simulink model "Observer_hoeksnelheidsmeter_SIU1"  (R2018b)
settings: Solver=FixedStepAuto  StartTime=0.0  StopTime=2  RelTol=1e-3
values from neighbouring files (symbols this model uses):
  A = [-(bm*(n^2) + bg)/(Jm*(n^2) + Jg) Kt*n/(Jm*(n^2) + Jg) ... (first row only)    [integratieTestScript.m]    (also in integratieTestScriptSIU2.m)
  B = [0 ... (first row only)    [integratieTestScript.m]    (also in integratieTestScriptSIU2.m)
  C = [1 0]    [integratieTestScript.m]    (also in integratieTestScriptSIU2.m)
  D = [0]    [integratieTestScript.m]    (also in integratieTestScriptSIU2.m)
  Kt = 0.083796    [integratieTestScript.m]
  n = 16.5    [integratieTestScript.m]
undefined symbols (not defined in the file or in its folder): DiscIntNeverNeededParam
libraries: simulink x2, dspswit3 x2, dspstat3 x1, peLuenbergerObserver x1, pePwmGenerator x1, powerlib_meascontrol x1
settings Model: Creator=Roberto  LastModifiedBy=Roberto

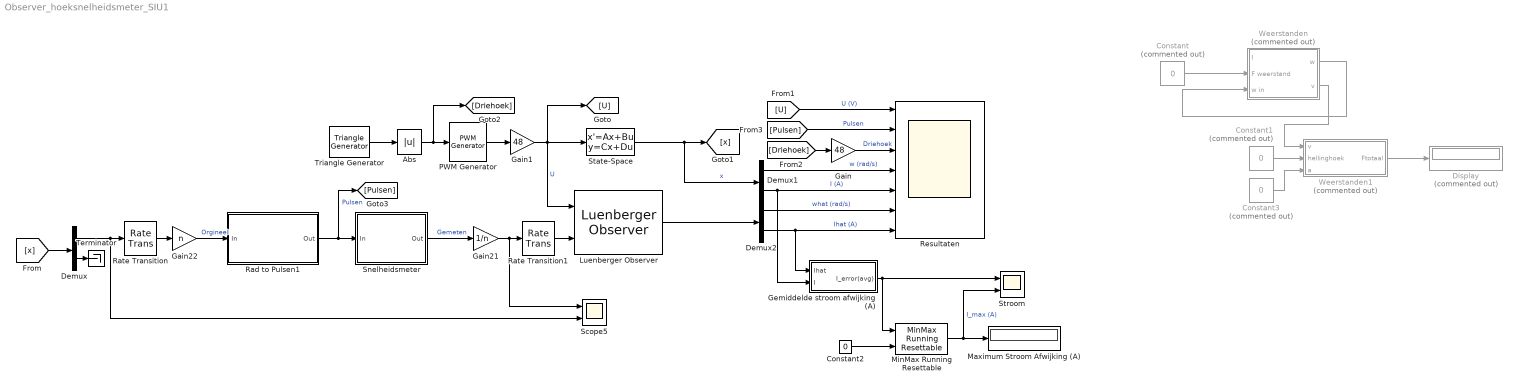
== system Observer_hoeksnelheidsmeter_SIU1 ==
  Abs : Abs
  Constant : Constant  Commented=on  Value=0
  Constant1 : Constant  Commented=on  Value=0
  Constant2 : Constant  Value=0
  Constant3 : Constant  Commented=on  Value=0
  Demux : Demux  Outputs=2
  Demux1 : Demux  Outputs=2
  Demux2 : Demux  Outputs=2
  Display : Display  Commented=on
  Gain : Gain  Gain=48
  Gain1 : Gain  Gain=48
  Gain21 : Gain  Gain=1/n
  Gain22 : Gain  Gain=n
  Gemiddelde stroom afwijking (A) : Subsystem
  Luenberger Observer : peLuenbergerObserver/Luenberger Observer  StateSpaceType=Continuous-time  Ad=Adh  Bd=Bdh  Cd=C  Dd=0  A=A  B=B  C=C  D=D  ObserverDesign=Observer gain  Ld=L  DesiredEigenvalues=eigenVal  x0=[0 0]  Tsd=0.1  Ts=1e-6
  Maximum Stroom Afwijking (A) : Display
  MinMax Running Resettable : simulink/Math Operations/MinMax Running Resettable  Function=max  vinit=0.0
  PWM Generator : pePwmGenerator/PWM Generator  CarrCount=Up  Tper=1/20000  Ts=1e-6
  Rad to Pulsen1 : Subsystem
  Rate Transition : RateTransition  OutPortSampleTime=1/100000
  Rate Transition1 : RateTransition  OutPortSampleTime=1e-6
  Resultaten : Scope  NumInputPorts=7
  Scope5 : Scope  NumInputPorts=2
  Snelheidsmeter : Subsystem
  State-Space : StateSpace  A=A  B=B  C=eye(2)  D=[0; 0]  InitialCondition=0
  Stroom : Scope  NumInputPorts=2
  Terminator : Terminator
  Triangle Generator : powerlib_meascontrol/Pulse & Signal Generators/Triangle Generator  Freq=0.5  Phase=90  Ts=1e-6
  Weerstanden : Subsystem  Commented=on
  Weerstanden1 : Subsystem  Commented=on
      mask init:
      | %% Parameter
      | 
      | %Mass'a
      | 
      | m = 2.067%130
      | 
      | g = 9.81
      | 
      | frol = 0.005
  wires:
  State-Space/1 -> Demux1/1, [x]  "x"
  Luenberger Observer/1 -> Demux2/1
  Gain22/1 -> Rad to Pulsen1/1(In)  "Orgineel"
  Snelheidsmeter/1(Out) -> Gain21/1  "Gemeten"
  Rad to Pulsen1/1(Out) -> [Pulsen], Snelheidsmeter/1(In)  "Pulsen"
  Demux/1 -> Scope5/2, Rate Transition/1
  Gain21/1 -> Scope5/1, Rate Transition1/1
  Rate Transition/1 -> Gain22/1
  Constant/1 -> Weerstanden/2(F weerstand)
  Weerstanden/1(w) -> Weerstanden/3(w in)
  Constant3/1 -> Weerstanden1/3(a)
  Constant1/1 -> Weerstanden1/2(hellinghoek)
  Weerstanden1/1(Ftotaal) -> Display/1
  Weerstanden/2(v) -> Weerstanden1/1(v)
  Rate Transition1/1 -> Luenberger Observer/2
  [x] -> Demux/1
  Demux/2 -> Terminator/1
  Constant2/1 -> MinMax Running Resettable/2
  MinMax Running Resettable/1 -> Stroom/2, Maximum Stroom Afwijking (A)/1  "I_max (A)"
  Gain/1 -> Resultaten/3  "Driehoek"
  [U] -> Resultaten/1  "U (V)"
  Demux2/1 -> Resultaten/6  "what (rad/s)"
  Demux2/2 -> Gemiddelde stroom afwijking (A)/1(Ihat), Resultaten/7  "Ihat (A)"
  [Driehoek] -> Gain/1
  Demux1/1 -> Resultaten/4  "w (rad/s)"
  Demux1/2 -> Gemiddelde stroom afwijking (A)/2(I), Resultaten/5  "I (A)"
  Gemiddelde stroom afwijking (A)/1(I_error(avg)) -> Stroom/1, MinMax Running Resettable/1
  Triangle Generator/1 -> Abs/1
  Abs/1 -> [Driehoek], PWM Generator/1
  Gain1/1 -> Luenberger Observer/1, [U], State-Space/1  "U"
  PWM Generator/1 -> Gain1/1
  [Pulsen] -> Resultaten/2  "Pulsen"

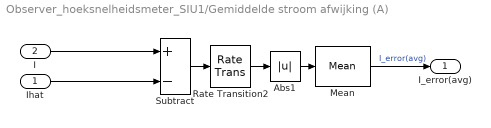
== system Observer_hoeksnelheidsmeter_SIU1/Gemiddelde stroom afwijking (A) ==
  Ihat : Inport
  I : Inport  Port=2
  Abs1 : Abs
  Mean : dspstat3/Mean  run=on  reset_popup=None  directionMode=Entire input  dimension=1  roiEnable=off  roiType=Rectangles  roiPortion=Entire ROI  roiOutput=Individual statistics for each ROI  roiFlag=off  roundingMode=Floor  overflowMode=off  outputDataTypeStr=Inherit: Same as accumulator  outputMin=[]  outputMax=[]  outputLastDataTypeStr=Inherit: Same as accumulator
  Rate Transition2 : RateTransition  OutPortSampleTime=1e-6
  Subtract : Sum  Inputs=+-
  I_error(avg) : Outport
  wires:
  I/1 -> Subtract/1
  Abs1/1 -> Mean/1
  Subtract/1 -> Rate Transition2/1
  Rate Transition2/1 -> Abs1/1
  Mean/1 -> I_error(avg)/1  "I_error(avg)"
  Ihat/1 -> Subtract/2

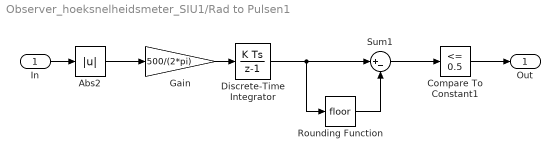
== system Observer_hoeksnelheidsmeter_SIU1/Rad to Pulsen1 ==
  In : Inport
  Abs2 : Abs
  Compare To Constant1 : simulink/Logic and Bit Operations/Compare To Constant  relop=<=  const=0.5  OutDataTypeStr=boolean
  Discrete-Time Integrator : DiscreteIntegrator  SampleTime=-1  ICPrevOutput=DiscIntNeverNeededParam  ICPrevScaledInput=DiscIntNeverNeededParam
  Gain : Gain  Gain=500/(2*pi)
  Rounding Function : Rounding
  Sum1 : Sum  Inputs=|+-
  Out : Outport
  wires:
  Rounding Function/1 -> Sum1/2
  Discrete-Time Integrator/1 -> Rounding Function/1, Sum1/1
  Compare To Constant1/1 -> Out/1
  Sum1/1 -> Compare To Constant1/1
  Gain/1 -> Discrete-Time Integrator/1
  In/1 -> Abs2/1
  Abs2/1 -> Gain/1

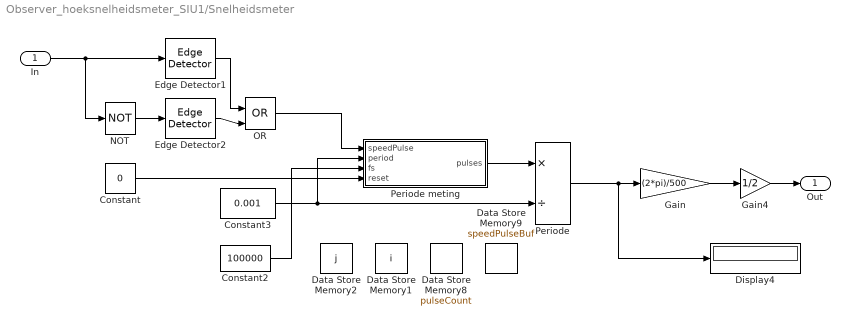
== system Observer_hoeksnelheidsmeter_SIU1/Snelheidsmeter ==
  In : Inport
  Constant : Constant  Value=0
  Constant2 : Constant  Value=100000
  Constant3 : Constant  Value=0.001
  Data Store Memory1 : DataStoreMemory  DataStoreName=i  ReadBeforeWriteMsg=warning  WriteAfterWriteMsg=warning  WriteAfterReadMsg=warning  InitialValue=1  ShowAdditionalParam=off  OutDataTypeStr=uint32
  Data Store Memory2 : DataStoreMemory  DataStoreName=j  ReadBeforeWriteMsg=warning  WriteAfterWriteMsg=warning  WriteAfterReadMsg=warning  InitialValue=2  ShowAdditionalParam=off  OutDataTypeStr=uint32
  Data Store Memory8 : DataStoreMemory  DataStoreName=pulseCount  ReadBeforeWriteMsg=warning  WriteAfterWriteMsg=warning  WriteAfterReadMsg=warning  ShowAdditionalParam=off  OutDataTypeStr=uint32
  Data Store Memory9 : DataStoreMemory  DataStoreName=speedPulseBuf  ReadBeforeWriteMsg=warning  WriteAfterWriteMsg=warning  WriteAfterReadMsg=warning  ShowAdditionalParam=off  OutDataTypeStr=uint8  Dimensions=10001
  Display4 : Display
  Edge Detector1 : dspswit3/Edge Detector  InputProcessing=Columns as channels (frame based)
      settings: SourceProductName=DSP System Toolbox  SourceProductBaseCode=DS
  Edge Detector2 : dspswit3/Edge Detector  InputProcessing=Columns as channels (frame based)
      settings: SourceProductName=DSP System Toolbox  SourceProductBaseCode=DS
  Gain : Gain  Gain=(2*pi)/500
  Gain4 : Gain  Gain=1/2
  NOT : Logic  Operator=NOT  IconShape=distinctive  AllPortsSameDT=off  OutDataTypeStr=boolean
  OR : Logic  Operator=OR  IconShape=distinctive  AllPortsSameDT=off  OutDataTypeStr=boolean
  Periode : Product  Inputs=*/
  Periode meting : MATLAB Function  TreatAsAtomicUnit=on
  Out : Outport
  wires:
  Constant3/1 -> Periode/2, Periode meting/2(period)
  Periode/1 -> Gain/1, Display4/1
  Constant2/1 -> Periode meting/3(fs)
  Periode meting/1(pulses) -> Periode/1
  In/1 -> NOT/1, Edge Detector1/1
  Gain/1 -> Gain4/1
  Constant/1 -> Periode meting/4(reset)
  OR/1 -> Periode meting/1(speedPulse)
  Edge Detector1/1 -> OR/1
  Edge Detector2/1 -> OR/2
  NOT/1 -> Edge Detector2/1
  Gain4/1 -> Out/1

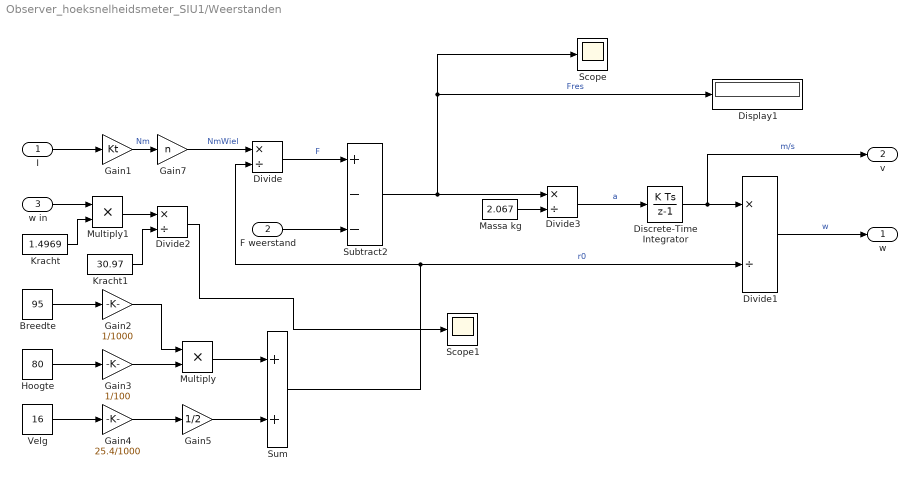
== system Observer_hoeksnelheidsmeter_SIU1/Weerstanden ==
  I : Inport
  F weerstand : Inport  Port=2
  w in : Inport  Port=3
  Breedte : Constant  Value=95
  Discrete-Time Integrator : DiscreteIntegrator  SampleTime=-1  ICPrevOutput=DiscIntNeverNeededParam  ICPrevScaledInput=DiscIntNeverNeededParam
  Display1 : Display
  Divide{,1..3} (4 alike) : Product  Inputs=*/
  Gain1 : Gain  Gain=Kt
  Gain2 : Gain  Gain=1/1000
  Gain3 : Gain  Gain=1/100
  Gain4 : Gain  Gain=25.4/1000
  Gain5 : Gain  Gain=1/2
  Gain7 : Gain  Gain=n
  Hoogte : Constant  Value=80
  Kracht : Constant  Value=1.4969
  Kracht1 : Constant  Value=30.97
  Massa kg : Constant  Value=2.067
  Multiply : Product
  Multiply1 : Product
  Scope : Scope
  Scope1 : Scope
  Subtract2 : Sum  Inputs=+--
  Sum : Sum
  Velg : Constant  Value=16
  w : Outport
  v : Outport  Port=2
  wires:
  Gain2/1 -> Multiply/1
  Discrete-Time Integrator/1 -> v/1, Divide1/1  "m/s"
  I/1 -> Gain1/1
  Subtract2/1 -> Scope/1, Display1/1, Divide3/1  "Fres"
  Massa kg/1 -> Divide3/2
  Gain4/1 -> Gain5/1
  Divide1/1 -> w/1  "w"
  Sum/1 -> Divide/2, Divide1/2  "r0"
  Gain3/1 -> Multiply/2
  Divide/1 -> Subtract2/1  "F"
  Multiply/1 -> Sum/1
  Gain5/1 -> Sum/2
  Hoogte/1 -> Gain3/1
  Breedte/1 -> Gain2/1
  Velg/1 -> Gain4/1
  Gain7/1 -> Divide/1  "NmWiel"
  Divide3/1 -> Discrete-Time Integrator/1  "a"
  Gain1/1 -> Gain7/1  "Nm"
  F weerstand/1 -> Subtract2/3
  w in/1 -> Multiply1/1
  Kracht/1 -> Multiply1/2
  Multiply1/1 -> Divide2/1
  Kracht1/1 -> Divide2/2
  Divide2/1 -> Scope1/1

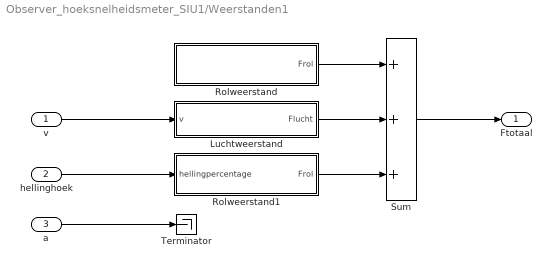
== system Observer_hoeksnelheidsmeter_SIU1/Weerstanden1 ==
  v : Inport
  hellinghoek : Inport  Port=2
  a : Inport  Port=3
  Luchtweerstand : Subsystem
  Rolweerstand : Subsystem
  Rolweerstand1 : Subsystem
  Sum : Sum  Inputs=+++
  Terminator : Terminator
  Ftotaal : Outport
  wires:
  v/1 -> Luchtweerstand/1(v)
  Sum/1 -> Ftotaal/1
  Rolweerstand/1(Frol) -> Sum/1
  Luchtweerstand/1(Flucht) -> Sum/2
  Rolweerstand1/1(Frol) -> Sum/3
  hellinghoek/1 -> Rolweerstand1/1(hellingpercentage)
  a/1 -> Terminator/1

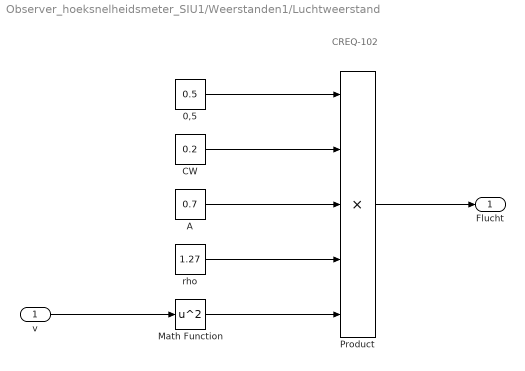
== system Observer_hoeksnelheidsmeter_SIU1/Weerstanden1/Luchtweerstand ==
  note: CREQ-102
  v : Inport
  0,5 : Constant  Value=0.5
  A : Constant  Value=0.7
  CW : Constant  Value=0.2
  Math Function : Math  Operator=square  RndMeth=Zero  SaturateOnIntegerOverflow=on
  Product : Product  Inputs=5
  rho : Constant  Value=1.27
  Flucht : Outport
  wires:
  Product/1 -> Flucht/1
  CW/1 -> Product/2
  A/1 -> Product/3
  0,5/1 -> Product/1
  rho/1 -> Product/4
  v/1 -> Math Function/1
  Math Function/1 -> Product/5

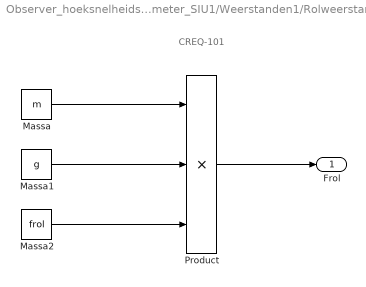
== system Observer_hoeksnelheidsmeter_SIU1/Weerstanden1/Rolweerstand ==
  note: CREQ-101
  Massa : Constant  Value=m
  Massa1 : Constant  Value=g
  Massa2 : Constant  Value=frol
  Product : Product  Inputs=3
  Frol : Outport
  wires:
  Massa/1 -> Product/1
  Massa2/1 -> Product/3
  Massa1/1 -> Product/2
  Product/1 -> Frol/1

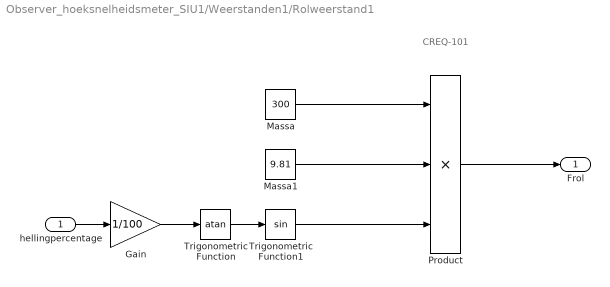
== system Observer_hoeksnelheidsmeter_SIU1/Weerstanden1/Rolweerstand1 ==
  note: CREQ-101
  hellingpercentage : Inport
  Gain : Gain  Gain=1/100
  Massa : Constant  Value=300
  Massa1 : Constant  Value=9.81
  Product : Product  Inputs=3
  Trigonometric Function : Trigonometry  Operator=atan
  Trigonometric Function1 : Trigonometry
  Frol : Outport
  wires:
  Product/1 -> Frol/1
  Massa1/1 -> Product/2
  Trigonometric Function1/1 -> Product/3
  Massa/1 -> Product/1
  hellingpercentage/1 -> Gain/1
  Gain/1 -> Trigonometric Function/1
  Trigonometric Function/1 -> Trigonometric Function1/1

== matlab function Observer_hoeksnelheidsmeter_SIU1/Snelheidsmeter/Periode meting ==
  data: speedPulse input; pulses output; speedPulseBuf data_store_memory; pulseCount data_store_memory; period input; i data_store_memory; fs input; j data_store_memory; reset input
function pulses = fcn(speedPulse,period, fs, reset)

global pulseCount;
global speedPulseBuf;
global i;
global j;

if reset == 1
    speedPulseBuf = uint8(zeros(size(speedPulseBuf)));
end

bufTime = period*fs + 1;

if i > bufTime
    i = uint32(1);
end

if j > bufTime
    j = uint32(1);
end

speedPulseBuf(i) = speedPulse;
pulseCount = pulseCount + uint32(speedPulse);
pulseCount = pulseCount - uint32(speedPulseBuf(j));

i = i + 1;
j = j + 1;

pulses = pulseCount;
